simulink model "pro1_wind"  (R2014b)
settings: Solver=ode3  StartTime=0.0  StopTime=10  FixedStep=0.001  RelTol=1e-3
libraries: powerlib x7, re_lib x1
settings Model: Creator=HPSEDC  LastModifiedBy=HPSEDC

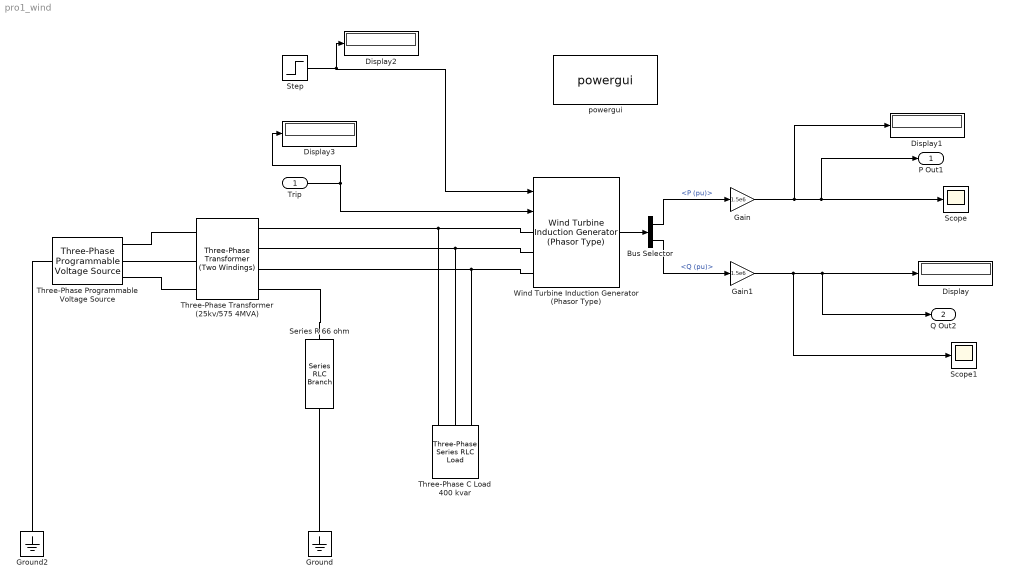
== system pro1_wind ==
  Trip : Inport
  Bus Selector : BusSelector  OutputSignals=P (pu),Q (pu)
  Display{,1..3} (4 alike) : Display
  Gain : Gain  Gain=1.5e6
  Gain1 : Gain  Gain=1.5e6
  Ground : powerlib/Elements/Ground  LConnTagsString=a
  Ground2 : powerlib/Elements/Ground  LConnTagsString=a
  Scope : Scope
      settings: TimeRange=30  YMin=-1  YMax=1  MaxDataPoints=10000
  Scope1 : Scope
      settings: TimeRange=30  YMin=-1  YMax=1
  "Series R 66 ohm  " : powerlib/Elements/Series RLC Branch  LConnTagsString=__new0  RConnTagsString=__new0  BranchType=R  Resistance=66  Inductance=1e-3  SetiL0=off  InitialCurrent=0  Capacitance=1e-6  Setx0=off  InitialVoltage=0  Measurements=None
  Step : Step  After=8  SampleTime=0
  Three-Phase C Load 400 kvar : powerlib/Elements/Three-Phase Series RLC Load  LConnTagsString=A|B|C  Configuration=Delta  NominalVoltage=575  NominalFrequency=60  ActivePower=0  InductivePower=0  CapacitivePower=400e3  Measurements=Branch voltages  LoadType=constant Z
  Three-Phase Programmable Voltage Source : powerlib/Electrical Sources/Three-Phase Programmable Voltage Source  PositiveSequence="[100  0 60]"  VariationEntity=None  VariationType=Table of time-amplitude pairs  VariationTypeAlt=Step  VariationStep=0.5  VariationRate=10  VariationMagnitude=0.3  VariationFrequency=2  VariationTiming=[1 2]  VariationPhaseA=off  Amplitudes=[1 0.8 1.2 1.0]  TimeValues=[0 0.1 0.15 0.2]  HarmonicGeneration=off  HarmonicA=[3 0.2 -25 0]  HarmonicB=[2 0.15 35 2]  Timing="[0.05  3]"  BusType=swing  Pref=0  Qref=0  Qmin=-inf  Qmax=inf
  Three-Phase Transformer (25kv/575 4MVA) : powerlib/Elements/Three-Phase Transformer (Two Windings)  Winding1Connection=Yg  UNITS=pu  NominalPower=[ 4e6 , 60 ]  Winding1=[ 25e3 , 0.025/30 , 0.025 ]  Winding2Connection=Yn  Winding2=[ 575 , 0.025/30 , 0.025 ]  SetSaturation=off  Rm=500  Lm=inf  Saturation=[ 0,0 ; 0.0024,1.2 ; 1.0,1.52 ]  Hysteresis=off  DataFile='hysteresis'  SetInitialFlux=off  InitialFluxes=[ 0.8 , -0.8 , 0.7 ]  Measurements=None  MoreParameters=off  BreakLoop=off  DataType=off  TransfoNumber=1
  Wind Turbine Induction Generator (Phasor Type) : re_lib/Wind Generation/Wind Turbine Induction Generator (Phasor Type)  ShowParameters=Turbine data  nom=[1.5e3 575 60]  sta=[ 0.004843 0.1248]  rot=[ 0.004377 0.1791]  Lm=6.77  mec=[5.04 0.01 3]  init="[ -0.01,0   0,0,0   0,0,0 ]"  ExternalTm=off  DisplayTurbChar=off  pitch_angle=0  Pmec=1.5e6  wind_base=12  P_wind_base=1  speed_nom=1  K_pitch_gain=[5 25]  pitch_max=45  pitch_rate=2
  powergui : powerlib/powergui  Priority=1  SimulationMode=Phasor  SolverType=Tustin/Backward Euler (TBE)  SampleTime=50e-6  frequency=60  SPID=off  DisableSnubberDevices=off  DisableRonSwitches=off  DisableVfSwitches=off  SwTol=0  DisplayEquations=off  Interpol=off  methode=off  Ts=100  frequencyindice=60  Pbase=10e6  ErrMax=1e-4  Iterations=50  UnitsV=V  UnitsW=W  FunctionMessages=off  echomessages=off  HookPort=off  EnableUseOfTLC=off  x0status=blocks  RestoreLinks=warning  ResistiveCurrentMeasurement=off  Frange=[0:2:500]  Ylog=off  Xlog=on  ShowGrid=off  save=off  variable=ZData  structure=0  ZoomFFT=off  StartTime=0.0  cycles=1  DisplayStyle=1  fundamental=60  FreqAxis=off  MaxFrequency=1000  frequencyindicesteady=1  RmsSteady=1  display=off
  P Out1 : Outport
  Q Out2 : Outport  Port=2
  wires:
  Wind Turbine Induction Generator (Phasor Type)/1 -> Bus Selector/1
  Bus Selector/2 -> Gain1/1  "<Q (pu)>"
  Bus Selector/1 -> Gain/1  "<P (pu)>"
  Gain/1 -> Display1/1, P Out1/1, Scope/1
  Gain1/1 -> Scope1/1, Display/1, Q Out2/1
  Trip/1 -> Wind Turbine Induction Generator (Phasor Type)/2, Display3/1
  Step/1 -> Wind Turbine Induction Generator (Phasor Type)/1, Display2/1
  connections:
  Three-Phase Programmable Voltage Source/RConn2 -- Three-Phase Transformer (25kv/575 4MVA)/LConn2
  Three-Phase Programmable Voltage Source/RConn1 -- Three-Phase Transformer (25kv/575 4MVA)/LConn1
  Three-Phase Programmable Voltage Source/RConn3 -- Three-Phase Transformer (25kv/575 4MVA)/LConn3
  Three-Phase Transformer (25kv/575 4MVA)/RConn1 -- Three-Phase C Load 400 kvar/LConn1 -- Wind Turbine Induction Generator (Phasor Type)/LConn1
  Three-Phase Transformer (25kv/575 4MVA)/RConn2 -- Three-Phase C Load 400 kvar/LConn2 -- Wind Turbine Induction Generator (Phasor Type)/LConn2
  Three-Phase Transformer (25kv/575 4MVA)/RConn3 -- Three-Phase C Load 400 kvar/LConn3 -- Wind Turbine Induction Generator (Phasor Type)/LConn3
  Three-Phase Transformer (25kv/575 4MVA)/RConn4 -- "Series R 66 ohm  "/LConn1
  Ground/LConn1 -- "Series R 66 ohm  "/RConn1
  Three-Phase Programmable Voltage Source/LConn1 -- Ground2/LConn1
